simulink model "EHSV_1st_stage"  (R2015a)
settings: Solver=ode45  StartTime=0.0  StopTime=10.0  RelTol=1e-3
undefined symbols (not defined in the file or in its folder): As_ehsv, K2_ehsv, Ki_ehsv, Kr_ehsv, ksi_ehsv, Kw_ehsv, w_n_ehsv
settings Model: Creator=HBALLEST  LastModifiedBy=Pedro H
settings OptimizationCC: ExpressionDepthLimit=2147483647
settings DebuggingCC: UnderspecifiedInitializationDetection=Classic  MergeDetectMultiDrivingBlocksExec=none  SolverPrmCheckMsg=warning  StateNameClashWarn=warning

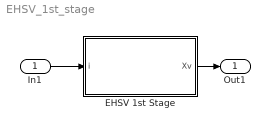
== system EHSV_1st_stage ==
  In1 : Inport
  EHSV 1st Stage : Subsystem
  Out1 : Outport
  wires:
  EHSV 1st Stage/1(Xv) -> Out1/1
  In1/1 -> EHSV 1st Stage/1(i)

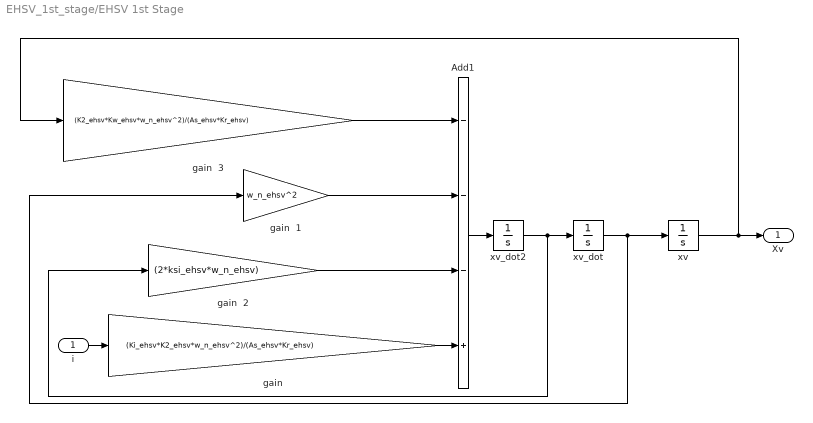
== system EHSV_1st_stage/EHSV 1st Stage ==
  i : Inport
  Add1 : Sum  Inputs=---+
  "gain  " : Gain  Gain=(Ki_ehsv*K2_ehsv*w_n_ehsv^2)/(As_ehsv*Kr_ehsv)
  gain  1 : Gain  Gain=w_n_ehsv^2
  gain  2 : Gain  Gain=(2*ksi_ehsv*w_n_ehsv)
  gain  3 : Gain  Gain=(K2_ehsv*Kw_ehsv*w_n_ehsv^2)/(As_ehsv*Kr_ehsv)
  xv : Integrator
  xv_dot : Integrator
  xv_dot2 : Integrator
  Xv : Outport
  wires:
  xv_dot/1 -> gain  1/1, xv/1
  xv_dot2/1 -> gain  2/1, xv_dot/1
  i/1 -> "gain  "/1
  Add1/1 -> xv_dot2/1
  xv/1 -> gain  3/1, Xv/1
  "gain  "/1 -> Add1/4
  gain  3/1 -> Add1/1
  gain  1/1 -> Add1/2
  gain  2/1 -> Add1/3
